simulink model "g1_p1_exp10_rl_bipolar"  (R2021b)
settings: Solver=ode45  StartTime=0.0  StopTime=0.5  RelTol=1e-3
libraries: spsMosfetLib x4, spsCurrentMeasurementLib x1, spsDCVoltageSourceLib x1, spsSeriesRLCBranchLib x1, spsTriangleGeneratorLib x1, spsVoltageMeasurementLib x1, spspowerguiLib x1
settings Model: Creator=marti  LastModifiedBy=marti
settings SolverCC: ZeroCrossAlgorithm=Adaptive
settings DebuggingCC: IgnoredZcDiagnostic=none

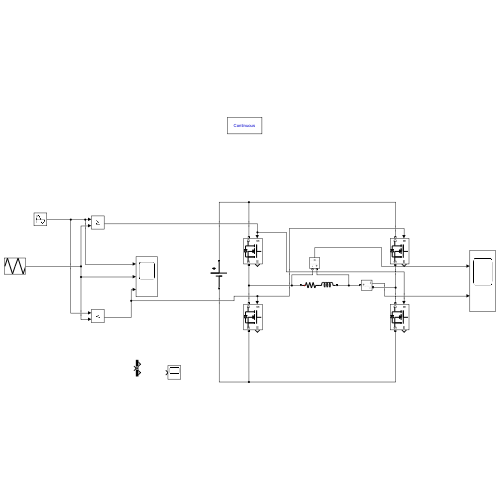
[thumbnail: Simulink's stored preview of the top-level diagram]
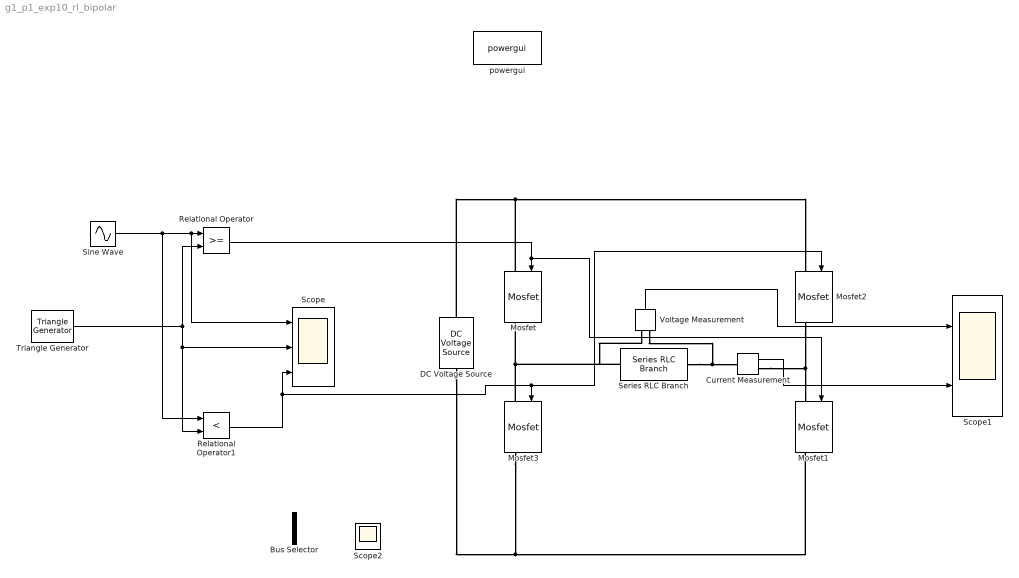
== system g1_p1_exp10_rl_bipolar ==
  Bus Selector : BusSelector  OutputSignals=signal1,signal2
  Current Measurement : spsCurrentMeasurementLib/Current Measurement  PhasorSimulation=off  OutputType=Complex  PSBequivalent=0
  DC Voltage Source : spsDCVoltageSourceLib/DC Voltage Source  Amplitude=100  Measurements=None
  Mosfet{,1..3} (4 alike) : spsMosfetLib/Mosfet  Ron=0.1  Lon=0  Rd=0.01  Vfd=0  IC=0  Rs=1e5  Cs=inf  Measurements=on
  Relational Operator : RelationalOperator  OutDataTypeStr=boolean  RndMeth=Simplest
  Relational Operator1 : RelationalOperator  Operator=<  OutDataTypeStr=boolean  RndMeth=Simplest
  Scope : Scope  NumInputPorts=3
  Scope1 : Scope  NumInputPorts=2
  Scope2 : Scope
  Series RLC Branch : spsSeriesRLCBranchLib/Series RLC Branch  LConnTagsString=__new0  RConnTagsString=__new0  BranchType=RL  Resistance=12.5  Inductance=6e-3  SetiL0=off  InitialCurrent=0  Capacitance=0  Setx0=off  InitialVoltage=0  Measurements=None
  Sine Wave : Sin  SampleTime=0
  Triangle Generator : spsTriangleGeneratorLib/Triangle Generator  Freq=1e3  Phase=90  Ts=0
  Voltage Measurement : spsVoltageMeasurementLib/Voltage Measurement  PhasorSimulation=off  OutputType=Complex  PSBequivalent=0
  powergui : spspowerguiLib/powergui  Priority=1  SimulationMode=Continuous  SampleTime=50e-6  frequency=60  Iterations=50  frequencyindice=0  Pbase=100e6  ErrMax=1e-4  UnitsV=kV  UnitsW=MW  buscounter=0  FunctionMessages=off  echomessages=off  EnableUseOfTLC=off  CurrentSourceSwitches=off  DisableSnubberDevices=off  DisableRonSwitches=off  DisableVfSwitches=off  DisplayEquations=off  AutomaticDiscreteSolvers=off  SolverType=Tustin/Backward Euler (TBE)  Interpol=off  ExternalGateDelay=off  methode=off  Ts=100  x0status=blocks  SPID=on  SwTol=0  HookPort=off  NonlinearTolerance=1e-4  nMaxIteration=100  ContinueOnMaxIteration=off  RestoreLinks=warning  ResistiveCurrentMeasurement=off  Frange=[0:2:500]  Ylog=off  Xlog=on  ShowGrid=off  save=off  variable=ZData  structure=0  ZoomFFT=off  StartTime=0.0  cycles=1  DisplayStyle=1  fundamental=60  FreqAxis=off  MaxFrequency=1000  frequencyindicesteady=1  RmsSteady=1  display=off
  wires:
  Relational Operator1/1 -> Scope/3, Mosfet2/1, Mosfet3/1
  Sine Wave/1 -> Relational Operator1/1, Scope/1, Relational Operator/1
  Triangle Generator/1 -> Scope/2, Relational Operator1/2, Relational Operator/2
  Relational Operator/1 -> Mosfet1/1, Mosfet/1
  Voltage Measurement/1 -> Scope1/1
  Current Measurement/1 -> Scope1/2
  connections:
  Mosfet3/LConn1 -- Voltage Measurement/LConn2 -- Series RLC Branch/LConn1 -- Mosfet/RConn1
  DC Voltage Source/RConn1 -- Mosfet/LConn1 -- Mosfet2/LConn1
  Mosfet2/RConn1 -- Mosfet1/LConn1 -- Current Measurement/RConn1
  Series RLC Branch/RConn1 -- Voltage Measurement/LConn1 -- Current Measurement/LConn1
  DC Voltage Source/LConn1 -- Mosfet3/RConn1 -- Mosfet1/RConn1
